simulink model "NaoLinearidadeAtuador"  (R2024a)
settings: Solver=FixedStepAuto  StartTime=0.0  StopTime=tf  FixedStep=step_modelo  RelTol=1e-3
undefined symbols (not defined in the file or in its folder): Td, Tpulse
settings Model: PacingRate=0.100000  Creator=rodri  LastModifiedBy=rodri
settings DataIOCC: SaveOutput=off  SaveTime=off
settings RTWCC: GPUComputeCapability=3.5

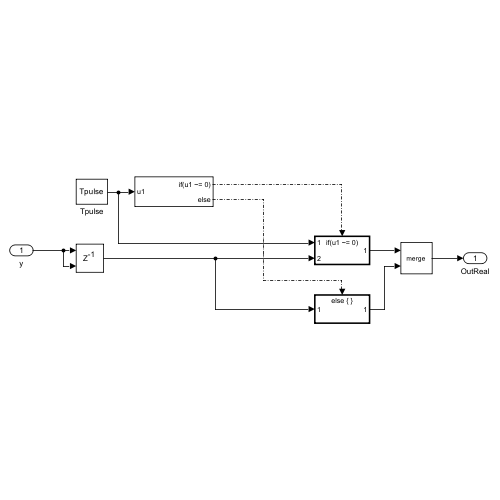
[thumbnail: Simulink's stored preview of the top-level diagram]
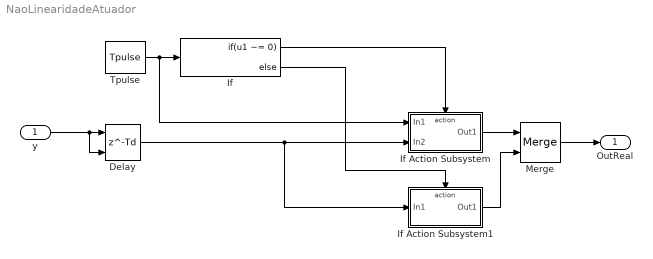
== system NaoLinearidadeAtuador ==
  y : Inport  OutDataTypeStr=double  PortDimensions=1
  Delay : Delay  DelayLength=Td  InitialConditionSource=Input port  InitialCondition=0
      settings: InputPortMap=u0,p4
  If : If  IfExpression=u1 ~= 0
  If Action Subsystem : Subsystem  TreatAsAtomicUnit=on
  If Action Subsystem1 : Subsystem  TreatAsAtomicUnit=on
  Merge : Merge
  Tpulse : Constant  Value=Tpulse  SampleTime=-1
  OutReal : Outport  OutDataTypeStr=double  PortDimensions=1
  wires:
  Tpulse/1 -> If Action Subsystem/1(In1), If/1
  y/1 -> Delay/2, Delay/1
  Delay/1 -> If Action Subsystem1/1(In1), If Action Subsystem/2(In2)
  Merge/1 -> OutReal/1
  If/1 -> If Action Subsystem/Action
  If/2 -> If Action Subsystem1/Action
  If Action Subsystem/1(Out1) -> Merge/1
  If Action Subsystem1/1(Out1) -> Merge/2

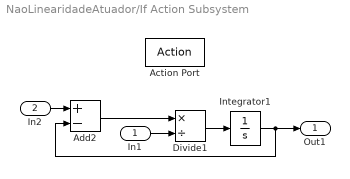
== system NaoLinearidadeAtuador/If Action Subsystem ==
  In1 : Inport
  In2 : Inport  Port=2
  Action Port : ActionPort  ActionPortLabel=if(u1 ~= 0)
  Add2 : Sum  Inputs=+-
  Divide1 : Product  Inputs=*/
  Integrator1 : Integrator
  Out1 : Outport
  wires:
  In2/1 -> Add2/1
  Integrator1/1 -> Out1/1, Add2/2
  Add2/1 -> Divide1/1
  Divide1/1 -> Integrator1/1
  In1/1 -> Divide1/2

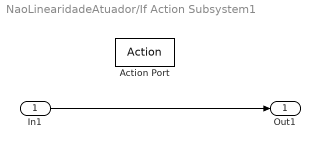
== system NaoLinearidadeAtuador/If Action Subsystem1 ==
  In1 : Inport
  Action Port : ActionPort  ActionPortLabel=else
  Out1 : Outport
  wires:
  In1/1 -> Out1/1
